simulink subsystem "Position_Controller_C"  (R2022b)
settings: Solver=VariableStepAuto  StartTime=0.0  StopTime=10.0  RelTol=1e-3
undefined symbols (not defined in the file or in its folder): conv, motor, Ri, Rw, sat
settings Model: Creator=gotta  LastModifiedBy=gotta

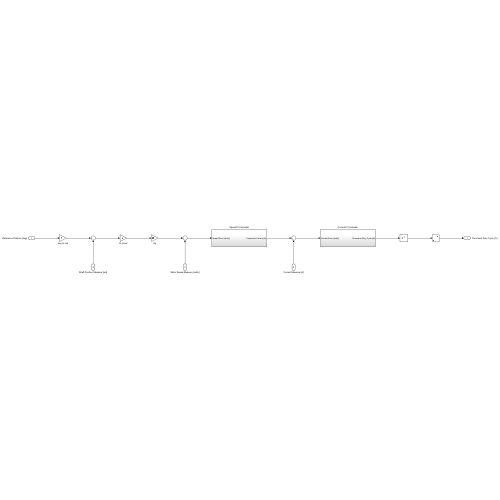
[thumbnail: Simulink's stored preview of the top-level diagram]
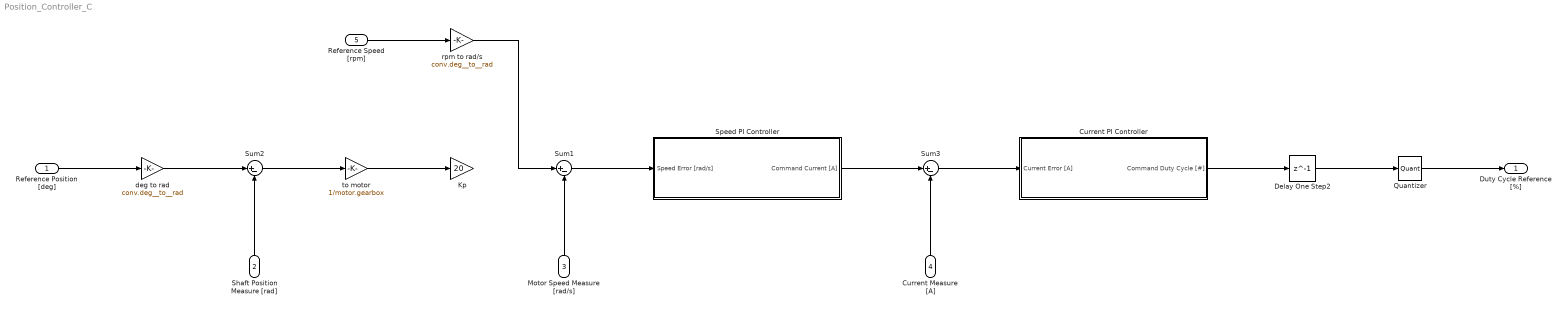
== system Position_Controller_C ==
  Reference Position [deg] : Inport
  Shaft Position Measure [rad] : Inport  Port=2
  Motor Speed Measure [rad/s] : Inport  Port=3
  Current Measure [A] : Inport  Port=4
  Reference Speed [rpm] : Inport  Port=5
  Current PI Controller : Subsystem
  Delay One Step2 : Delay  DelayLength=1
  Kp : Gain  Gain=20
  Quantizer : Quantizer  QuantizationInterval=uc.duty_step
  Speed PI Controller : Subsystem
  Sum1 : Sum  Inputs=|+-
  Sum2 : Sum  Inputs=|+-
  Sum3 : Sum  Inputs=|+-
  deg to rad : Gain  Gain=conv.deg__to__rad
  rpm to rad/s : Gain  Gain=conv.deg__to__rad
  to motor : Gain  Gain=1/motor.gearbox
  Duty Cycle Reference [%] : Outport
  wires:
  Reference Position [deg]/1 -> deg to rad/1
  Speed PI Controller/1(Command Current [A]) -> Sum3/1
  Quantizer/1 -> Duty Cycle Reference [%]/1
  Motor Speed Measure [rad/s]/1 -> Sum1/2
  Sum3/1 -> Current PI Controller/1(Current Error [A])
  Delay One Step2/1 -> Quantizer/1
  Current Measure [A]/1 -> Sum3/2
  Sum1/1 -> Speed PI Controller/1(Speed Error [rad/s])
  to motor/1 -> Kp/1
  Current PI Controller/1(Command Duty Cycle [#]) -> Delay One Step2/1
  deg to rad/1 -> Sum2/1
  Shaft Position Measure [rad]/1 -> Sum2/2
  Sum2/1 -> to motor/1
  Reference Speed [rpm]/1 -> rpm to rad/s/1
  rpm to rad/s/1 -> Sum1/1

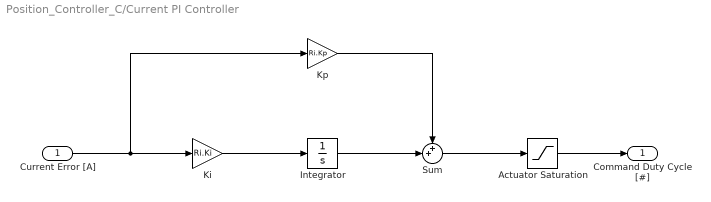
== system Position_Controller_C/Current PI Controller ==
  Current Error [A] : Inport
  Actuator Saturation : Saturate  UpperLimit=sat.d  LowerLimit=-sat.d
  Integrator : Integrator  LimitOutput=on  UpperSaturationLimit=sat.d  LowerSaturationLimit=-sat.d
  Ki : Gain  Gain=Ri.Ki
  Kp : Gain  Gain=Ri.Kp
  Sum : Sum  Inputs=++|
  Command Duty Cycle [#] : Outport
  wires:
  Integrator/1 -> Sum/2
  Ki/1 -> Integrator/1
  Sum/1 -> Actuator Saturation/1
  Kp/1 -> Sum/1
  Current Error [A]/1 -> Ki/1, Kp/1
  Actuator Saturation/1 -> Command Duty Cycle [#]/1

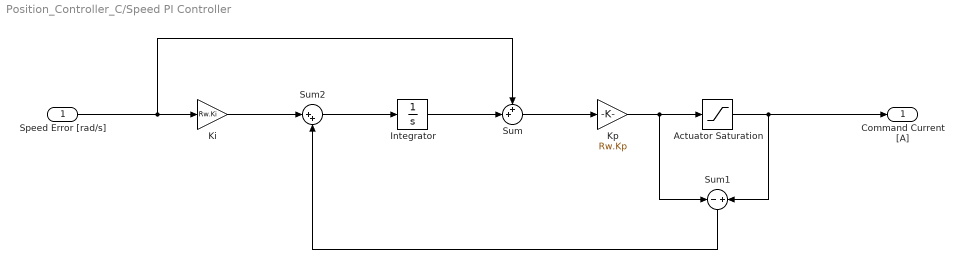
== system Position_Controller_C/Speed PI Controller ==
  Speed Error [rad/s] : Inport
  Actuator Saturation : Saturate  UpperLimit=sat.I  LowerLimit=-sat.I
  Integrator : Integrator  LimitOutput=on  UpperSaturationLimit=sat.I  LowerSaturationLimit=-sat.I
  Ki : Gain  Gain=Rw.Ki
  Kp : Gain  Gain=Rw.Kp
  Sum : Sum  Inputs=++|
  Sum1 : Sum  Inputs=-+
  Sum2 : Sum  Inputs=|++
  Command Current [A] : Outport
  wires:
  Integrator/1 -> Sum/2
  Sum/1 -> Kp/1
  Ki/1 -> Sum2/1
  Sum2/1 -> Integrator/1
  Sum1/1 -> Sum2/2
  Kp/1 -> Actuator Saturation/1, Sum1/1
  Speed Error [rad/s]/1 -> Sum/1, Ki/1
  Actuator Saturation/1 -> Command Current [A]/1, Sum1/2
